simulink model "test_toggling_led_complete_behavior"  (R2022b)
settings: Solver=FixedStepDiscrete  StartTime=0.0  StopTime=10  FixedStep=0.1  RelTol=1e-3  EnableMultiTasking=on
settings Model: Creator=cristian  LastModifiedBy=cristian
settings SolverCC: AlgebraicLoopSolver=TrustRegion  AutoInsertRateTranBlk=on
settings DataIOCC: LimitDataPoints=on
settings OptimizationCC: LifeSpan=inf
settings DebuggingCC: UnconnectedInputMsg=warning  UnconnectedOutputMsg=warning  UnconnectedLineMsg=warning  AllowSymbolicDim=off  SFUnexpectedBacktrackingDiag=warning  SFNoUnconditionalDefaultTransitionDiag=warning  SFExecutionAtInitializationDiag=none  ArithmeticOperatorsInVariantConditions=warning
settings ModelReferenceCC: EnableRefExpFcnMdlSchedulingChecks=on
settings SFSimCC: SimUseLocalCustomCode=off  CustomCodeUndefinedFunction=UseInterfaceOnly
settings RTWCC: RTWUseLocalCustomCode=off  DLArmComputeVersion=19.05
settings CodeAppCC: StateflowObjectComments=on
settings GRTTargetCC: TargetLangStandard=C89/C90 (ANSI)
settings ConfigComp: CovMetricSettings=dw  CovSaveCumulativeToWorkspaceVar=on  CovSaveSingleToWorkspaceVar=on  CovExternalEMLEnable=off  CovSFcnEnable=off  DVTestSuiteOptimization=Auto  DVDetectOutOfBounds=on  DVModelReferenceHarness=on  DVHarnessSource=Signal Editor

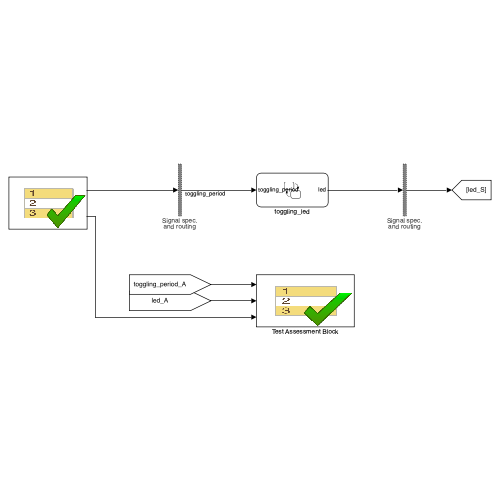
[thumbnail: Simulink's stored preview of the top-level diagram]
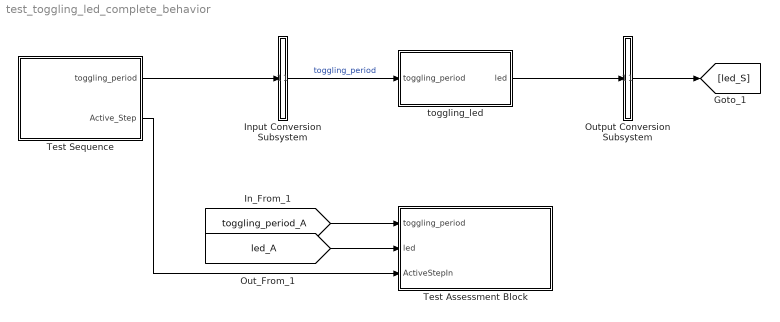
== system test_toggling_led_complete_behavior ==
  Input Conversion Subsystem : Subsystem  Tag=__SLT_ICS__  Description=|
      | Signal spec.
      | and routing
      settings: AttributesFormatString=%<Description>
  Output Conversion Subsystem : Subsystem  Tag=__SLT_OCS__  Description=|
      | Signal spec.
      | and routing
      settings: AttributesFormatString=%<Description>
  Test Assessment Block : Test Sequence  Tag=__SLT_ASMT__  TreatAsAtomicUnit=on
  Test Sequence : Test Sequence  TreatAsAtomicUnit=on
  toggling_led : Stateflow chart  TreatAsAtomicUnit=on
  wires:
  [toggling_period_A] -> Test Assessment Block/1(toggling_period)
  [led_A] -> Test Assessment Block/2(led)
  Test Sequence/1(toggling_period) -> Input Conversion Subsystem/1(Inport_1)
  Output Conversion Subsystem/1(Outport_1) -> [led_S]
  Input Conversion Subsystem/1(Outport_1) -> toggling_led/1(toggling_period)  "toggling_period"
  toggling_led/1(led) -> Output Conversion Subsystem/1(Inport_1)
  Test Sequence/2(Active_Step) -> Test Assessment Block/3(ActiveStepIn)

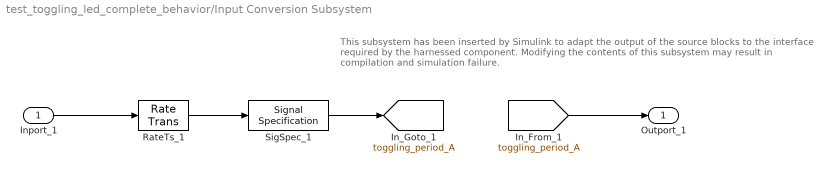
== system test_toggling_led_complete_behavior/Input Conversion Subsystem ==
  note: This subsystem has been inserted by Simulink to adapt the output of the source blocks to the interface required by the harnessed component.
      |  Modifying the contents of this subsystem may result in compilation and simulation failure.
  Inport_1 : Inport
  RateTs_1 : RateTransition  OutPortSampleTime=0.1
  SigSpec_1 : SignalSpecification  OutDataTypeStr=double  Dimensions=[1]  SampleTime=0.1
  Outport_1 : Outport
  tag scope: toggling_period_A=global
  wires:
  [toggling_period_A] -> Outport_1/1
  SigSpec_1/1 -> [toggling_period_A]
  RateTs_1/1 -> SigSpec_1/1
  Inport_1/1 -> RateTs_1/1

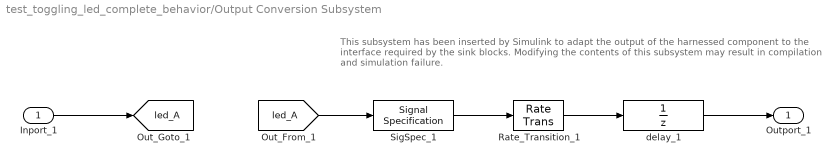
== system test_toggling_led_complete_behavior/Output Conversion Subsystem ==
  note: This subsystem has been inserted by Simulink to adapt the output of the harnessed component to the interface required by the sink blocks.
      |  Modifying the contents of this subsystem may result in compilation and simulation failure.
  Inport_1 : Inport
  Rate_Transition_1 : RateTransition  OutPortSampleTimeOpt=Inherit
  SigSpec_1 : SignalSpecification  OutDataTypeStr=boolean  Dimensions=[1]  SampleTime=0.1
  delay_1 : UnitDelay  SampleTime=-1
  Outport_1 : Outport
  tag scope: led_A=global
  wires:
  Inport_1/1 -> [led_A]
  [led_A] -> SigSpec_1/1
  SigSpec_1/1 -> Rate_Transition_1/1
  Rate_Transition_1/1 -> delay_1/1
  delay_1/1 -> Outport_1/1

== stateflow chart test_toggling_led_complete_behavior/Test Assessment Block ==
  state CompleteBehavior
    state Run
      state Verify_CB_Init
        verify(led == 0);
      state Verify_CB_Period1
        state Verify_CB_Period1_1
          verify(led == 1);
        state Verify_CB_Period1_2
          verify(led == 0);
        (default) -> Verify_CB_Period1_1
        Verify_CB_Period1_1 -> Verify_CB_Period1_2 : [
            | after(toggling_period,sec)
            | ]
      state Verify_CB_Period2
        state Verify_CB_Period2_1
          verify(led == 1);
        state Verify_CB_Period2_2
          verify(led == 0);
        (default) -> Verify_CB_Period2_1
        Verify_CB_Period2_1 -> Verify_CB_Period2_2 : [
            | after(toggling_period,sec)
            | ]
      state Verify_CB_Reset1
        verify(led == 0);
      state Verify_CB_Period3
        verify(led == 1);
      state Verify_CB_Reset2
        verify(led == 0);
      state Run_1
      Run -> (junction 257)
      (default) -> (junction 257)
      (junction 257) -> (junction 258) [order 1] : [ActiveStepIn == ActiveStepEnumH4.CB_Init
          | ]
      (junction 258) -> Verify_CB_Init [order 1] : [~in(CompleteBehavior.Run.Verify_CB_Init)]
      (junction 257) -> (junction 266) [order 2]
      (junction 258) -> (junction 261) [order 2]
      (junction 266) -> (junction 267) [order 1] : [ActiveStepIn == ActiveStepEnumH4.CB_Period1
          | ]
      (junction 267) -> Verify_CB_Period1 [order 1] : [~in(CompleteBehavior.Run.Verify_CB_Period1)]
      (junction 266) -> (junction 280) [order 2]
      (junction 267) -> (junction 270) [order 2]
      (junction 280) -> (junction 281) [order 1] : [ActiveStepIn == ActiveStepEnumH4.CB_Period2
          | ]
      (junction 281) -> Verify_CB_Period2 [order 1] : [~in(CompleteBehavior.Run.Verify_CB_Period2)]
      (junction 280) -> (junction 294) [order 2]
      (junction 281) -> (junction 284) [order 2]
      (junction 294) -> (junction 295) [order 1] : [ActiveStepIn == ActiveStepEnumH4.CB_Reset1
          | ]
      (junction 295) -> Verify_CB_Reset1 [order 1] : [~in(CompleteBehavior.Run.Verify_CB_Reset1)]
      (junction 294) -> (junction 302) [order 2]
      (junction 295) -> (junction 298) [order 2]
      (junction 302) -> (junction 303) [order 1] : [ActiveStepIn == ActiveStepEnumH4.CB_Period3
          | ]
      (junction 303) -> Verify_CB_Period3 [order 1] : [~in(CompleteBehavior.Run.Verify_CB_Period3)]
      (junction 302) -> (junction 310) [order 2]
      (junction 303) -> (junction 306) [order 2]
      (junction 310) -> (junction 311) [order 1] : [ActiveStepIn == ActiveStepEnumH4.CB_Reset2
          | ]
      (junction 311) -> Verify_CB_Reset2 [order 1] : [~in(CompleteBehavior.Run.Verify_CB_Reset2)]
      (junction 311) -> (junction 314) [order 2]
      (junction 318) -> (junction 319)
      (junction 319) -> Run_1 [order 1] : [~in(CompleteBehavior.Run.Run_1)]
      (junction 319) -> (junction 322) [order 2]
      (junction 310) -> (junction 318) [order 2]
    (default) -> Run
  (default) -> CompleteBehavior : {assert(Active_Scenario_Index == 1,'The value of Scenario Parameter ''Active_Scenario_Index'' is not valid. Use the index of the scenario to specify it.')}
  data: toggling_period input double size=[1]; led input boolean size=[1]; ActiveStepIn input; Active_Scenario_Index parameter =1

== stateflow chart test_toggling_led_complete_behavior/toggling_led ==
  note: Lo spegnimento ha invece la priorità, appena ho periodo=0 spengo.
  state Off
    en: led = LOW
  state Blink_Off
    en:
    led = LOW
    period = toggling_period
  state Blink_On
    en:
    led = HIGH
    period = toggling_period
  note: L'utilizzo di una variabile di appoggio consente di gestire il caso in cui durante il blinking il periodo viene cambiato. Usando tale variabile, lo stato corrente viene termianto dopo un'attesa pari al vecchio periodo e dal nuovo stato vi sarà la variazione di periodo.
      | Ad esempio, se passo da 1s a 2s, ed attualmente il led è acceso, lo spegnerò terminando l'attesa di 1s e dal prossimo stato l'attesa sarà di 2s.
  (default) -> Off
  Blink_Off -> Off [order 1] : [toggling_period == 0]
  Blink_On -> Off [order 1] : [toggling_period == 0]
  Off -> Blink_On : [toggling_period ~= 0]
  Blink_On -> Blink_Off [order 2] : [after(period,sec)]
  Blink_Off -> Blink_On [order 2] : [after(period,sec)]
  data: toggling_period input double; led output boolean; HIGH constant boolean =1; LOW constant boolean =0; period local

== stateflow chart test_toggling_led_complete_behavior/Test Sequence ==
  settings: updateMethod=DISCRETE  sampleTime=0.1
  state CompleteBehavior
    state CB_Init
      %% Initialize data outputs.
      toggling_period = 0;
      settings: description=Partiamo da un periodo nullo, quindi il led non si accende mai.
    state CB_Period1
      toggling_period = 1;
      settings: description=Impostiamo un peridoo di 1.
    state CB_Period2
      toggling_period = 2;
      settings: description=Impostiamo un periodo di 2.
    state CB_Reset1
      toggling_period = 0;
      settings: description=Spegniamo il led.
    state CB_Period3
      toggling_period = 0.5;
      settings: description=Impostiamo un periodo minore di 1.
    state CB_Reset2
      toggling_period = 0;
      settings: description=Spegniamo definitivamente.
    (default) -> CB_Init
    CB_Init -> CB_Period1 : [
        | after(1,sec)
        | ]
    CB_Period1 -> CB_Period2 : [
        | after(toggling_period*2,sec)
        | ]
    CB_Period2 -> CB_Reset1 : [
        | after(toggling_period*2,sec)
        | ]
    CB_Reset1 -> CB_Period3 : [
        | true
        | ]
    CB_Period3 -> CB_Reset2 : [
        | after(toggling_period,sec)
        | ]
  (default) -> CompleteBehavior : {assert(Active_Scenario_Index == 1,'The value of Scenario Parameter ''Active_Scenario_Index'' is not valid. Use the index of the scenario to specify it.')}
  data: toggling_period output double size=[1]; Active_Step output Enum: ActiveStepEnumH4; Active_Scenario_Index parameter =1
